simulink library "library"  (R2020a)
settings: Solver=VariableStepAuto  StartTime=0.0  StopTime=10.0  RelTol=1e-3
values from neighbouring files (symbols this model uses):
  height = 1080    [setup.m]    (also in setupSystem.m = heightName(nameIdx))
  nRho = maxRho*2    [setup.m]    (also in setupSystem.m)
  theta = (0:dTheta:180-dTheta)    [ARLHT.m]    (also in setup.m = (0:1:179); setupSystem.m = (0:1:179))
  width = 1920    [setup.m]    (also in setupSystem.m = widthName(nameIdx))
libraries: simulink x135, hdlsllib x83, $bdroot x15
(part 1 of 3)
settings Model: Creator=david  LastModifiedBy=david

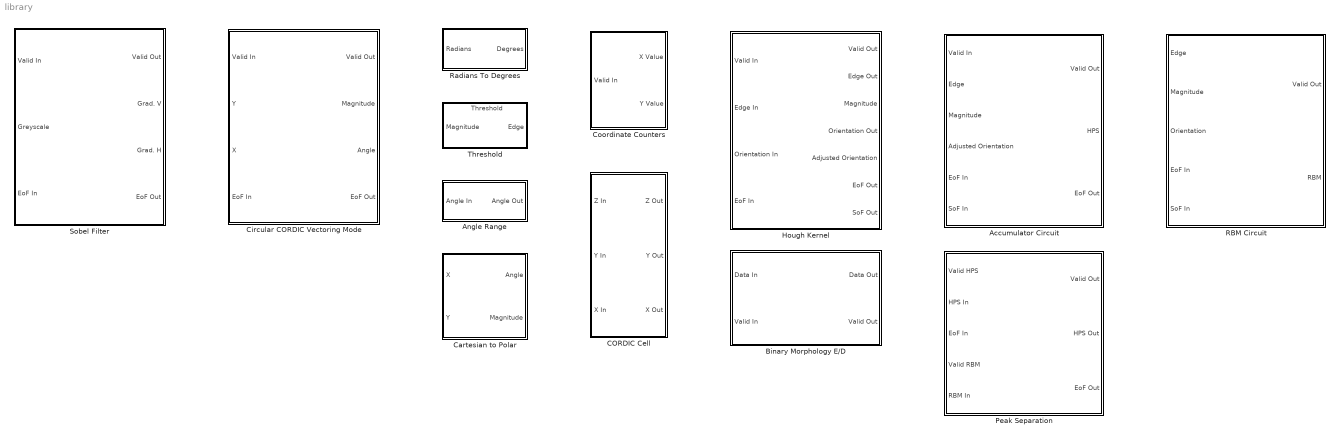
== system library ==
  Accumulator Circuit : Subsystem  mask{height=height, width=width, rhoBits=ceil(log2(ceil(sqrt(height^2+width^2)*4))), nTheta=length(theta), nRho=nRho}
      mask prompts: height "Image Height:"; width "Image Width:"; rhoBits "Address Bits:"; nTheta "Number Theta:"; nRho "Number Rho:"
      mask init:
      | kTheta = 4;
  Angle Range : Subsystem
  Binary Morphology E/D : Subsystem  mask{operation=Erosion, height=height, width=width}
      mask prompts: height "Image Height:"; width "Image Width:"
      mask init:
      | if get_param(gcb, 'operation') == "Erosion"
      |     op = 0;
      | else
      |     op = 1;
      | end
      mask TypeOptions operation: Erosion | Dilation
      mask DialogControl ParameterGroupVar Prompt: Main
  CORDIC Cell : Subsystem  mask{k=0}
      mask prompts: k "Iteration Number:"
  Cartesian to Polar : Subsystem  mask{b=16, f=8}
      mask prompts: b "Angle Wordlength:"; f "Angle Fractional Bits:"
      mask DialogControl DescGroupVar Prompt: Cartesian to Polar
      mask DialogControl DescTextVar Prompt: Convert cartesian coordinates to polar representation. This block uses Circular CORDIC operating in vectoring mode. The output angle is in the range [-90, 90] degrees.
      mask DialogControl ParameterGroupVar Prompt: Main
  Circular CORDIC Vectoring Mode : Subsystem  mask{i=12, b=24, f=13}
      mask prompts: i "Number of Iterations:"; b "Wordlength:"; f "Fractional Bits:"
      mask DialogControl DescGroupVar Prompt: Circular CORDIC Vectoring Mode
      mask DialogControl DescTextVar Prompt: Implements circular CORDIC operating in vectoring mode. Outputs magnitude of x and y inputs. Computes the angle in range [-pi, pi].
      mask DialogControl ParameterGroupVar Prompt: Main
  Coordinate Counters : Subsystem  mask{height=480, width=640}
      mask prompts: height "Image Height:"; width "Image Width:"
      mask DialogControl DescGroupVar Prompt: Coordinate Counters
      mask DialogControl DescTextVar Prompt: Coordinate HDL counters to keep track of coordinate values.
      mask DialogControl ParameterGroupVar Prompt: Main
  Hough Kernel : Subsystem  mask{rhoBits=ceil(log2(ceil(sqrt(height^2+width^2))*2)), height=height, width=width, dTheta=1}
      mask prompts: rhoBits "Address Bits:"; height "Image Height:"; width "Image Width:"; dTheta "Theta Resolution:"
      mask init:
      | kTheta = 4;
      | maxRho = ceil(sqrt((height/2)^2+(width/2)^2));
      | theta = (0:dTheta:180-dTheta);
      | gamma = (theta(end) + dTheta)/kTheta;
  Peak Separation : Subsystem  mask{nRho=ceil(sqrt(height^2+width^2))*2, nTheta=length(theta)}
      mask prompts: nRho "HPS Height:"; nTheta "HPS Width:"
      mask DialogControl DescGroupVar Prompt: Peak Separation
      mask DialogControl ParameterGroupVar Prompt: Main
  RBM Circuit : Subsystem  mask{height=height, width=width, nTheta=length(theta), rhoBits=ceil(log2(ceil(sqrt(height^2+width^2))*2)), nRho=nRho}
      mask prompts: height "Image Height:"; width "Image Width:"; nTheta "Number Theta:"; rhoBits "Address Bits:"; nRho "Number Rho:"
  Radians To Degrees : Subsystem  mask{f=0}
      mask prompts: f "Fractional Bits:"
      mask DialogControl DescGroupVar Prompt: Radian to Degrees
      mask DialogControl DescTextVar Prompt: Convert radians to degrees and output angle based on input resolution in degrees.
      mask DialogControl ParameterGroupVar Prompt: Main
  Sobel Filter : Subsystem  mask{height=height, width=width}
      mask prompts: height "Image Height:"; width "Image Width:"
      mask DialogControl DescGroupVar Prompt: Sobel Filter
      mask DialogControl DescTextVar Prompt: The Sobel Filter block applies the Sobel edge detection filters to a greyscale image to produce the horizontal and vertical gradients. The symmetric border management scheme is used in this block.
      mask DialogControl ParameterGroupVar Prompt: Main
  Threshold : Subsystem  mask{b=11, f=0, s=0}
      mask prompts: b "Wordlength:"; f "Fractional Bits:"; s "Signed:"
      settings: PortSchema="{\"entries\":[{\"content\":{\"sides\":[{\"content\":{\"connectorIds\":[\"In1\"]},\"type\":\"ConnectorPlacement.EquallySpacedRectSide\",\"uuid\":\"2eddfc8d-913f-4b03-9e43-0dfa341f5c16\"},{\"content\":{\"connectorIds\":[\"Out1\"],\"side\":\"RIGHT\"},\"type\":\"ConnectorPlacement.EquallySpacedRectSide\",\"uuid\":\"673922c3-77d1-427d-93a1-c0d3defe75f8\"},{\"content\":{\"connectorIds\":[\"In2\"],\"side\":\"TOP\"},\"type\":\"ConnectorPlacement.EquallySpacedRectSide\",\"uuid\":\"7679a1c8-69e5-4154-8188-f484296a7f7e\"}]},\"type\":\"ConnectorPlacement.EquallySpacedConnector\",\"uuid\":\"713163ba-a4f5-4467-a1a5-cd71dca6c6a2\"}],\"packageUris\":[\"http://schema.mathworks.com/mf0/Connector/19700101\"],\"version\":\"1.0\"}"
      mask DialogControl DescGroupVar Prompt: Threshold
      mask DialogControl DescTextVar Prompt: Segment an input signal using a threshold value.
      mask DialogControl ParameterGroupVar Prompt: Main

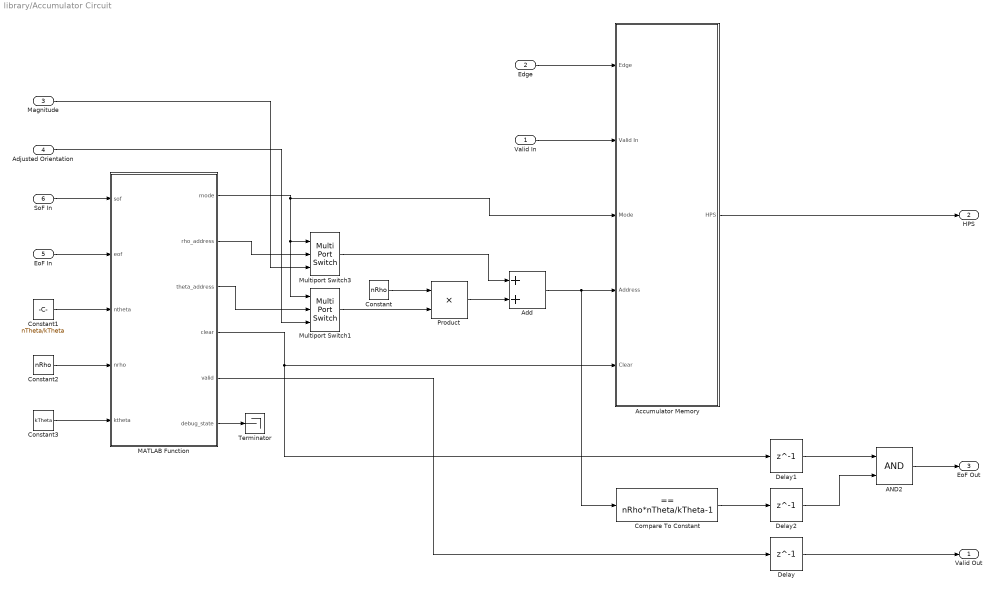
== system library/Accumulator Circuit ==
  Valid In : Inport
  Edge : Inport  Port=2
  Magnitude : Inport  Port=3
  Adjusted Orientation : Inport  Port=4
  EoF In : Inport  Port=5
  SoF In : Inport  Port=6
  AND2 : Logic  IconShape=distinctive  AllPortsSameDT=off  OutDataTypeStr=boolean
  Accumulator Memory : Subsystem
  Add : Sum  OutDataTypeStr=fixdt(0,ceil(log2(nRho*nTheta/kTheta)),0)
  Compare To Constant : simulink/Logic and Bit Operations/Compare To Constant  relop===  const=nRho*nTheta/kTheta-1  OutDataTypeStr=boolean
  Constant : Constant  Value=nRho  OutDataTypeStr=fixdt(0,ceil(log2(nRho+1)),0)  SampleTime=-1
  Constant1 : Constant  Value=nTheta/kTheta  OutDataTypeStr=uint8  SampleTime=-1
  Constant2 : Constant  Value=nRho  OutDataTypeStr=uint16  SampleTime=-1
  Constant3 : Constant  Value=kTheta  OutDataTypeStr=uint8  SampleTime=-1
  Delay : Delay  DelayLength=1  InitialCondition=0  UseCircularBuffer=on
  Delay1 : Delay  DelayLength=1  InitialCondition=0  UseCircularBuffer=on
  Delay2 : Delay  DelayLength=1  InitialCondition=0  UseCircularBuffer=on
  MATLAB Function : MATLAB Function  TreatAsAtomicUnit=on
  Multiport Switch1 : MultiPortSwitch  DataPortOrder=Zero-based contiguous  Inputs=2  zeroidx=on
  Multiport Switch3 : MultiPortSwitch  DataPortOrder=Zero-based contiguous  Inputs=2  zeroidx=on
  Product : Product  OutDataTypeStr=fixdt(0,ceil(log2(nRho*(nTheta/kTheta-1))),0)
  Terminator : Terminator
  Valid Out : Outport
  HPS : Outport  Port=2
  EoF Out : Outport  Port=3
  wires:
  EoF In/1 -> MATLAB Function/2(eof)
  MATLAB Function/3(theta_address) -> Multiport Switch1/2
  MATLAB Function/2(rho_address) -> Multiport Switch3/2
  MATLAB Function/1(mode) -> Accumulator Memory/3(Mode), Multiport Switch3/1, Multiport Switch1/1
  Constant/1 -> Product/1
  Product/1 -> Add/2
  Multiport Switch3/1 -> Add/1
  Multiport Switch1/1 -> Product/2
  Add/1 -> Accumulator Memory/4(Address), Compare To Constant/1
  Accumulator Memory/1(HPS) -> HPS/1
  Valid In/1 -> Accumulator Memory/2(Valid In)
  Edge/1 -> Accumulator Memory/1(Edge)
  Adjusted Orientation/1 -> Multiport Switch1/3
  Magnitude/1 -> Multiport Switch3/3
  Compare To Constant/1 -> Delay2/1
  Constant3/1 -> MATLAB Function/5(ktheta)
  Constant2/1 -> MATLAB Function/4(nrho)
  Constant1/1 -> MATLAB Function/3(ntheta)
  Delay2/1 -> AND2/2
  Delay1/1 -> AND2/1
  AND2/1 -> EoF Out/1
  Delay/1 -> Valid Out/1
  MATLAB Function/5(valid) -> Delay/1
  MATLAB Function/4(clear) -> Accumulator Memory/5(Clear), Delay1/1
  SoF In/1 -> MATLAB Function/1(sof)
  MATLAB Function/6(debug_state) -> Terminator/1

== system library/Angle Range ==
  Angle In : Inport
  Add : Sum  OutDataTypeStr=uint8
  Compare To Constant : simulink/Logic and Bit Operations/Compare To Constant  relop=<  const=0  OutDataTypeStr=boolean
  Constant : Constant  Value=180  OutDataTypeStr=uint8  SampleTime=-1
  Data Type Conversion : DataTypeConversion  OutDataTypeStr=uint8
  Multiport Switch : MultiPortSwitch  DataPortOrder=Zero-based contiguous  Inputs=2  zeroidx=on
  Angle Out : Outport
  wires:
  Constant/1 -> Add/2
  Add/1 -> Multiport Switch/3
  Data Type Conversion/1 -> Multiport Switch/2
  Compare To Constant/1 -> Multiport Switch/1
  Angle In/1 -> Compare To Constant/1, Data Type Conversion/1, Add/1
  Multiport Switch/1 -> Angle Out/1

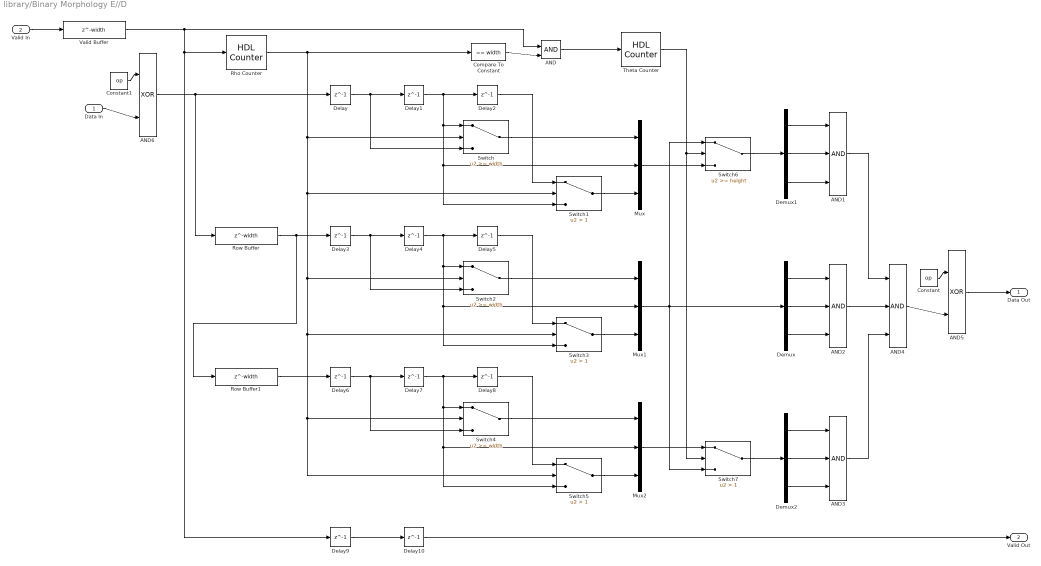
== system library/Binary Morphology E//D ==
  Data In : Inport
  Valid In : Inport  Port=2
  AND : Logic  IconShape=distinctive  AllPortsSameDT=off  OutDataTypeStr=boolean
  AND{1..4} (4 alike) : Logic  Inputs=3  IconShape=distinctive  AllPortsSameDT=off  OutDataTypeStr=boolean
  AND5 : Logic  Operator=XOR  IconShape=distinctive  AllPortsSameDT=off  OutDataTypeStr=boolean
  AND6 : Logic  Operator=XOR  IconShape=distinctive  AllPortsSameDT=off  OutDataTypeStr=boolean
  Compare To Constant : simulink/Logic and Bit Operations/Compare To Constant  relop===  const=width  OutDataTypeStr=boolean
  Constant : Constant  Value=op  OutDataTypeStr=Inherit: Inherit via back propagation  SampleTime=-1
  Constant1 : Constant  Value=op  OutDataTypeStr=Inherit: Inherit via back propagation  SampleTime=-1
  Delay{,1..10} (11 alike) : Delay  DelayLength=1
  Demux : Demux  Outputs=3
  Demux1 : Demux  Outputs=3
  Demux2 : Demux  Outputs=3
  Mux : Mux  Inputs=3
  Mux1 : Mux  Inputs=3
  Mux2 : Mux  Inputs=3
  Rho Counter : hdlsllib/Sources/HDL Counter  CountType=Count limited  CountInit=1  CountStep=1  CountMax=width  CountFromType=Initial value  CountFrom=1  CountResetPort=off  CountLoadPort=off  CountEnbPort=on  CountDirPort=off  CountDataType=Unsigned  CountWordLen=ceil(log2(width+1))  CountFracLen=0  CountSampTime=1
  Row Buffer : Delay  DelayLength=width
  Row Buffer1 : Delay  DelayLength=width
  Switch : Switch  Threshold=width
  Switch{1,3,5,7} (4 alike) : Switch  Criteria=u2 > Threshold  Threshold=1
  Switch2 : Switch  Threshold=width
  Switch4 : Switch  Threshold=width
  Switch6 : Switch  Threshold=height
  Theta Counter : hdlsllib/Sources/HDL Counter  CountType=Count limited  CountInit=1  CountStep=1  CountMax=height  CountFromType=Initial value  CountFrom=1  CountResetPort=off  CountLoadPort=off  CountEnbPort=on  CountDirPort=off  CountDataType=Unsigned  CountWordLen=ceil(log2(height+1))  CountFracLen=0  CountSampTime=1
  Valid Buffer : Delay  DelayLength=width
  Data Out : Outport
  Valid Out : Outport  Port=2
  wires:
  Data In/1 -> AND6/2
  AND6/1 -> Delay/1, Row Buffer/1
  Constant1/1 -> AND6/1
  Constant/1 -> AND5/1
  AND4/1 -> AND5/2
  AND3/1 -> AND4/3
  AND1/1 -> AND4/1
  AND2/1 -> AND4/2
  Demux2/3 -> AND3/3
  Demux2/1 -> AND3/1
  Demux2/2 -> AND3/2
  Demux/3 -> AND2/3
  Demux/2 -> AND2/2
  Demux/1 -> AND2/1
  Demux1/3 -> AND1/3
  Demux1/1 -> AND1/1
  Demux1/2 -> AND1/2
  Switch7/1 -> Demux2/1
  Mux2/1 -> Switch7/1
  Mux/1 -> Switch6/3
  Theta Counter/1 -> Switch6/2, Switch7/2
  Switch6/1 -> Demux1/1
  Mux1/1 -> Demux/1, Switch6/1, Switch7/3
  Row Buffer1/1 -> Delay6/1
  Rho Counter/1 -> Compare To Constant/1, Switch/2, Switch1/2, Switch2/2, Switch5/2, Switch4/2, Switch3/2
  Switch5/1 -> Mux2/3
  Switch4/1 -> Mux2/1
  Delay8/1 -> Switch5/1
  Delay7/1 -> Switch4/1, Switch5/3, Mux2/2, Delay8/1
  Delay6/1 -> Delay7/1, Switch4/3
  Delay3/1 -> Switch2/3, Delay4/1
  Delay4/1 -> Delay5/1, Mux1/2, Switch3/3, Switch2/1
  Delay5/1 -> Switch3/1
  Switch2/1 -> Mux1/1
  Switch3/1 -> Mux1/3
  Row Buffer/1 -> Row Buffer1/1, Delay3/1
  Switch1/1 -> Mux/3
  Switch/1 -> Mux/1
  Delay2/1 -> Switch1/1
  Delay1/1 -> Switch/1, Switch1/3, Mux/2, Delay2/1
  Delay/1 -> Delay1/1, Switch/3
  Compare To Constant/1 -> AND/2
  AND/1 -> Theta Counter/1
  Valid In/1 -> Valid Buffer/1
  Valid Buffer/1 -> Rho Counter/1, Delay9/1, AND/1
  Delay9/1 -> Delay10/1
  Delay10/1 -> Valid Out/1
  AND5/1 -> Data Out/1

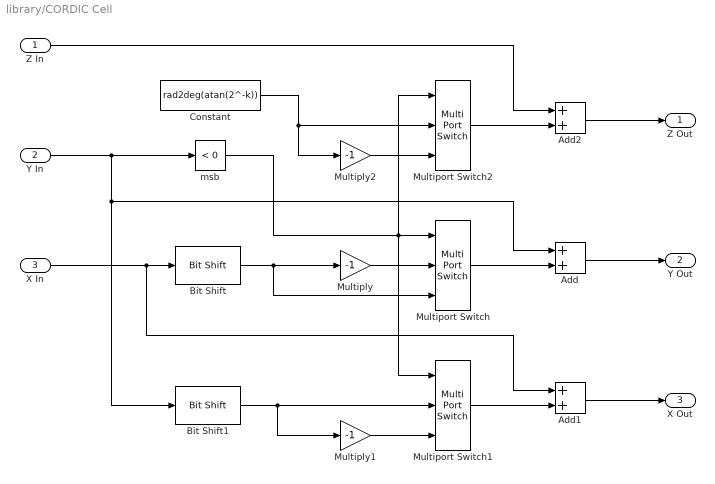
== system library/CORDIC Cell ==
  Z In : Inport
  Y In : Inport  Port=2
  X In : Inport  Port=3
  Add : Sum  RndMeth=Round  SaturateOnIntegerOverflow=on  OutDataTypeStr=Inherit: Same as first input
  Add1 : Sum  RndMeth=Round  SaturateOnIntegerOverflow=on  OutDataTypeStr=Inherit: Same as first input
  Add2 : Sum  RndMeth=Round  SaturateOnIntegerOverflow=on  OutDataTypeStr=Inherit: Same as first input
  Bit Shift : hdlsllib/Logic and Bit Operations/Bit Shift  mode=Shift Right Arithmetic  N=k
  Bit Shift1 : hdlsllib/Logic and Bit Operations/Bit Shift  mode=Shift Right Arithmetic  N=k
  Constant : Constant  Value=rad2deg(atan(2^-k))  OutDataTypeStr=Inherit: Inherit via back propagation  SampleTime=-1
  Multiply : Gain  Gain=-1  OutDataTypeStr=Inherit: Same as input
  Multiply1 : Gain  Gain=-1  OutDataTypeStr=Inherit: Same as input
  Multiply2 : Gain  Gain=-1  OutDataTypeStr=Inherit: Same as input
  Multiport Switch : MultiPortSwitch  DataPortOrder=Zero-based contiguous  Inputs=2  zeroidx=on
  Multiport Switch1 : MultiPortSwitch  DataPortOrder=Zero-based contiguous  Inputs=2  zeroidx=on
  Multiport Switch2 : MultiPortSwitch  DataPortOrder=Zero-based contiguous  Inputs=2  zeroidx=on
  msb : simulink/Logic and Bit Operations/Compare To Constant  relop=<  const=0  OutDataTypeStr=boolean
  Z Out : Outport
  Y Out : Outport  Port=2
  X Out : Outport  Port=3
  wires:
  Multiply1/1 -> Multiport Switch1/3
  Multiply/1 -> Multiport Switch/2
  Add/1 -> Y Out/1
  Add1/1 -> X Out/1
  Add2/1 -> Z Out/1
  Multiport Switch/1 -> Add/2
  Multiport Switch1/1 -> Add1/2
  X In/1 -> Bit Shift/1, Add1/1
  Bit Shift1/1 -> Multiply1/1, Multiport Switch1/2
  Bit Shift/1 -> Multiply/1, Multiport Switch/3
  msb/1 -> Multiport Switch/1, Multiport Switch1/1, Multiport Switch2/1
  Y In/1 -> msb/1, Bit Shift1/1, Add/1
  Z In/1 -> Add2/1
  Multiply2/1 -> Multiport Switch2/3
  Constant/1 -> Multiply2/1, Multiport Switch2/2
  Multiport Switch2/1 -> Add2/2

== system library/Cartesian to Polar ==
  X : Inport
  Y : Inport  Port=2
  CORDIC Cells : Subsystem
  Compare To Zero : simulink/Logic and Bit Operations/Compare To Zero  relop=~=  OutDataTypeStr=boolean
  Gain : Gain  Gain=1/1.6467  ParamDataTypeStr=fixdt(0,16,16)  RndMeth=Round  SaturateOnIntegerOverflow=on  OutDataTypeStr=Inherit: Same as input
  Multiport Switch : MultiPortSwitch  DataPortOrder=Zero-based contiguous  Inputs=2  zeroidx=on
  Quadrant Demapper : Subsystem
  Quadrant Mapper : Subsystem
  Terminator : Terminator
  Z : Constant  Value=0  OutDataTypeStr=fixdt(1,b,f)  SampleTime=-1
  Angle : Outport
  Magnitude : Outport  Port=2
  wires:
  Quadrant Demapper/1(Z Out) -> Multiport Switch/3
  Multiport Switch/1 -> Angle/1
  Y/1 -> Quadrant Mapper/1(Y In)
  X/1 -> Quadrant Mapper/2(X In)
  Gain/1 -> Magnitude/1
  Compare To Zero/1 -> Multiport Switch/1
  CORDIC Cells/1(Z Out) -> Quadrant Demapper/1(Z In)
  Quadrant Mapper/3(Decision) -> Quadrant Demapper/2(Decision)
  CORDIC Cells/2(Y Out) -> Terminator/1
  CORDIC Cells/3(X Out) -> Gain/1
  Z/1 -> CORDIC Cells/1(Z In), Multiport Switch/2
  Quadrant Mapper/2(X Out) -> CORDIC Cells/3(X In)
  Quadrant Mapper/1(Y Out) -> CORDIC Cells/2(Y In), Compare To Zero/1

== system library/Circular CORDIC Vectoring Mode ==
  Valid In : Inport
  Y : Inport  Port=2
  X : Inport  Port=3
  EoF In : Inport  Port=4
  Cartesian to Polar : $bdroot/Cartesian to Polar  b=16  f=8
  Data Type Conversion : DataTypeConversion  OutDataTypeStr=fixdt(1,24,11)
  Data Type Conversion1 : DataTypeConversion  OutDataTypeStr=fixdt(1,24,11)
  Valid Out : Outport  VectorParamsAs1DForOutWhenUnconnected=off
  Magnitude : Outport  Port=2  VectorParamsAs1DForOutWhenUnconnected=off
  Angle : Outport  Port=3  VectorParamsAs1DForOutWhenUnconnected=off
  EoF Out : Outport  Port=4  VectorParamsAs1DForOutWhenUnconnected=off
  wires:
  Valid In/1 -> Valid Out/1
  Cartesian to Polar/1 -> Angle/1
  Cartesian to Polar/2 -> Magnitude/1
  EoF In/1 -> EoF Out/1
  X/1 -> Data Type Conversion/1
  Y/1 -> Data Type Conversion1/1
  Data Type Conversion/1 -> Cartesian to Polar/1
  Data Type Conversion1/1 -> Cartesian to Polar/2

== system library/Coordinate Counters ==
  Valid In : Inport
  AND : Logic  IconShape=distinctive  AllPortsSameDT=off  OutDataTypeStr=boolean
  Compare To Constant : simulink/Logic and Bit Operations/Compare To Constant  relop===  const=width/2-1  OutDataTypeStr=boolean
  X Counter : hdlsllib/Sources/HDL Counter  CountType=Count limited  CountInit=-width/2  CountStep=1  CountMax=width/2-1  CountFromType=Initial value  CountFrom=-width/2  CountResetPort=off  CountLoadPort=off  CountEnbPort=on  CountDirPort=off  CountDataType=Signed  CountWordLen=ceil(log2(width/2)) + 1  CountFracLen=0  CountSampTime=1
  Y Counter : hdlsllib/Sources/HDL Counter  CountType=Count limited  CountInit=-height/2  CountStep=1  CountMax=height/2-1  CountFromType=Initial value  CountFrom=-height/2  CountResetPort=off  CountLoadPort=off  CountEnbPort=on  CountDirPort=off  CountDataType=Signed  CountWordLen=ceil(log2(height/2)) + 1  CountFracLen=0  CountSampTime=1
  X Value : Outport  VectorParamsAs1DForOutWhenUnconnected=off
  Y Value : Outport  Port=2  VectorParamsAs1DForOutWhenUnconnected=off
  wires:
  Valid In/1 -> AND/2, X Counter/1
  X Counter/1 -> X Value/1, Compare To Constant/1
  Y Counter/1 -> Y Value/1
  AND/1 -> Y Counter/1
  Compare To Constant/1 -> AND/1

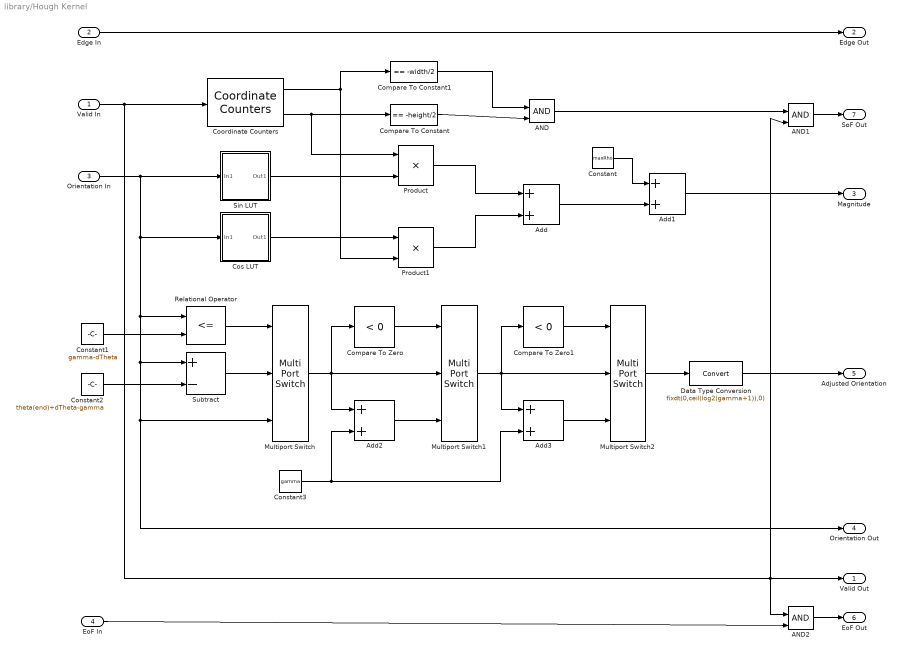
== system library/Hough Kernel ==
  Valid In : Inport
  Edge In : Inport  Port=2
  Orientation In : Inport  Port=3
  EoF In : Inport  Port=4
  AND : Logic  IconShape=distinctive  AllPortsSameDT=off  OutDataTypeStr=boolean
  AND1 : Logic  IconShape=distinctive  AllPortsSameDT=off  OutDataTypeStr=boolean
  AND2 : Logic  IconShape=distinctive  AllPortsSameDT=off  OutDataTypeStr=boolean
  Add : Sum
  Add1 : Sum  OutDataTypeStr=fixdt(0,rhoBits,0)
  Add2 : Sum  OutDataTypeStr=Inherit: Same as first input
  Add3 : Sum  OutDataTypeStr=Inherit: Same as first input
  Compare To Constant : simulink/Logic and Bit Operations/Compare To Constant  relop===  const=-height/2  OutDataTypeStr=boolean
  Compare To Constant1 : simulink/Logic and Bit Operations/Compare To Constant  relop===  const=-width/2  OutDataTypeStr=boolean
  Compare To Zero : simulink/Logic and Bit Operations/Compare To Zero  relop=<  OutDataTypeStr=boolean
  Compare To Zero1 : simulink/Logic and Bit Operations/Compare To Zero  relop=<  OutDataTypeStr=boolean
  Constant : Constant  Value=maxRho  OutDataTypeStr=fixdt(0,ceil(log2(maxRho+1)),0)  SampleTime=-1
  Constant1 : Constant  Value=gamma-dTheta  OutDataTypeStr=fixdt(0,ceil(log2(gamma)),0)  SampleTime=-1
  Constant2 : Constant  Value=theta(end)+dTheta-gamma  OutDataTypeStr=fixdt(0,ceil(log2(179+1-gamma)),0)  SampleTime=-1
  Constant3 : Constant  Value=gamma  OutDataTypeStr=fixdt(0,ceil(log2(gamma+1)),0)  SampleTime=-1
  Coordinate Counters : $bdroot/Coordinate Counters  height=height  width=width
  Cos LUT : Subsystem
  Data Type Conversion : DataTypeConversion  OutDataTypeStr=fixdt(0,ceil(log2(gamma+1)),0)
  Multiport Switch : MultiPortSwitch  DataPortOrder=Zero-based contiguous  Inputs=2  zeroidx=on
  Multiport Switch1 : MultiPortSwitch  DataPortOrder=Zero-based contiguous  Inputs=2  zeroidx=on
  Multiport Switch2 : MultiPortSwitch  DataPortOrder=Zero-based contiguous  Inputs=2  zeroidx=on
  Product : Product  OutDataTypeStr=fixdt(1,ceil(log2(height)),0)  RndMeth=Round
  Product1 : Product  OutDataTypeStr=fixdt(1,ceil(log2(width)),0)  RndMeth=Round
  Relational Operator : RelationalOperator  Operator=<=  OutDataTypeStr=boolean  RndMeth=Simplest
  Sin LUT : Subsystem
  Subtract : Sum  Inputs=+-  OutDataTypeStr=fixdt(1,9,0)
  Valid Out : Outport
  Edge Out : Outport  Port=2
  Magnitude : Outport  Port=3
  Orientation Out : Outport  Port=4
  Adjusted Orientation : Outport  Port=5
  EoF Out : Outport  Port=6
  SoF Out : Outport  Port=7
  wires:
  Edge In/1 -> Edge Out/1
  Coordinate Counters/2 -> Product/1, Compare To Constant/1
  Coordinate Counters/1 -> Product1/2, Compare To Constant1/1
  Product1/1 -> Add/2
  Constant/1 -> Add1/1
  Relational Operator/1 -> Multiport Switch/1
  Add/1 -> Add1/2
  Constant3/1 -> Add3/2, Add2/2
  Constant2/1 -> Subtract/2
  Add3/1 -> Multiport Switch2/3
  Add2/1 -> Multiport Switch1/3
  Add1/1 -> Magnitude/1
  Subtract/1 -> Multiport Switch/2
  Product/1 -> Add/1
  Compare To Zero1/1 -> Multiport Switch2/1
  Multiport Switch/1 -> Add2/1, Compare To Zero/1, Multiport Switch1/2
  Multiport Switch1/1 -> Add3/1, Compare To Zero1/1, Multiport Switch2/2
  Compare To Zero/1 -> Multiport Switch1/1
  Orientation In/1 -> Sin LUT/1(In1), Cos LUT/1(In1), Multiport Switch/3, Orientation Out/1, Subtract/1, Relational Operator/1
  Multiport Switch2/1 -> Data Type Conversion/1
  Constant1/1 -> Relational Operator/2
  Data Type Conversion/1 -> Adjusted Orientation/1
  Compare To Constant1/1 -> AND/1
  Compare To Constant/1 -> AND/2
  AND1/1 -> SoF Out/1
  AND/1 -> AND1/1
  Valid In/1 -> AND2/1, AND1/2, Valid Out/1, Coordinate Counters/1
  AND2/1 -> EoF Out/1
  EoF In/1 -> AND2/2
  Cos LUT/1(Out1) -> Product1/1
  Sin LUT/1(Out1) -> Product/2

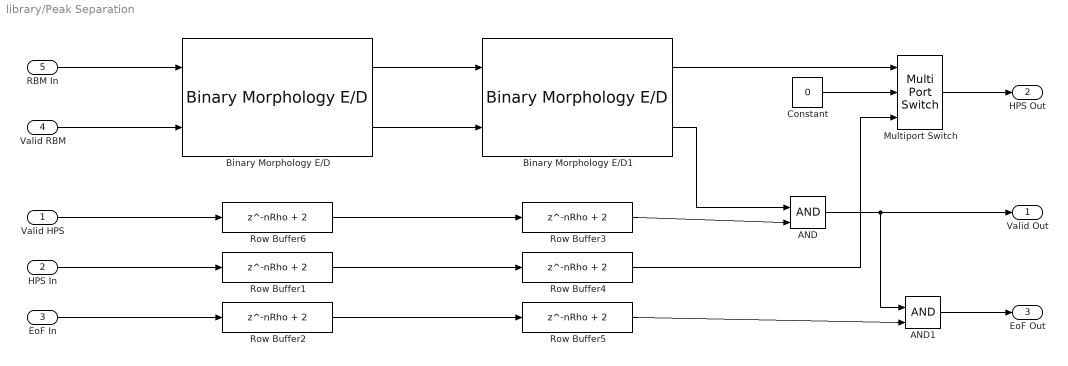
== system library/Peak Separation ==
  Valid HPS : Inport
  HPS In : Inport  Port=2
  EoF In : Inport  Port=3
  Valid RBM : Inport  Port=4
  RBM In : Inport  Port=5
  AND : Logic  IconShape=distinctive  AllPortsSameDT=off  OutDataTypeStr=boolean
  AND1 : Logic  IconShape=distinctive  AllPortsSameDT=off  OutDataTypeStr=boolean
  Binary Morphology E/D : $bdroot/Binary Morphology E//D  operation=Erosion  height=nTheta  width=nRho
  Binary Morphology E/D1 : $bdroot/Binary Morphology E//D  operation=Dilation  height=nTheta  width=nRho
  Constant : Constant  Value=0  OutDataTypeStr=Inherit: Inherit via back propagation  SampleTime=-1
  Multiport Switch : MultiPortSwitch  DataPortOrder=Zero-based contiguous  Inputs=2  zeroidx=on
  Row Buffer{1..6} (6 alike) : Delay  DelayLength=nRho + 2
  Valid Out : Outport
  HPS Out : Outport  Port=2
  EoF Out : Outport  Port=3
  wires:
  Row Buffer6/1 -> Row Buffer3/1
  Row Buffer2/1 -> Row Buffer5/1
  Row Buffer1/1 -> Row Buffer4/1
  Constant/1 -> Multiport Switch/2
  Row Buffer3/1 -> AND/2
  Binary Morphology E/D1/2 -> AND/1
  Valid HPS/1 -> Row Buffer6/1
  HPS In/1 -> Row Buffer1/1
  EoF In/1 -> Row Buffer2/1
  RBM In/1 -> Binary Morphology E/D/1
  Valid RBM/1 -> Binary Morphology E/D/2
  Binary Morphology E/D/1 -> Binary Morphology E/D1/1
  Binary Morphology E/D/2 -> Binary Morphology E/D1/2
  Binary Morphology E/D1/1 -> Multiport Switch/1
  Row Buffer4/1 -> Multiport Switch/3
  Multiport Switch/1 -> HPS Out/1
  AND1/1 -> EoF Out/1
  AND/1 -> AND1/1, Valid Out/1
  Row Buffer5/1 -> AND1/2

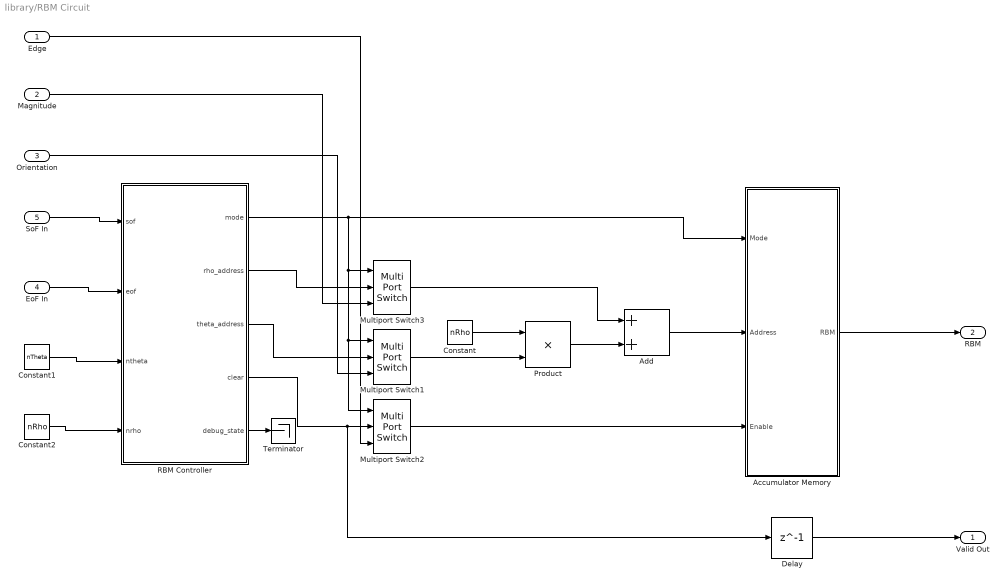
== system library/RBM Circuit ==
  Edge : Inport
  Magnitude : Inport  Port=2
  Orientation : Inport  Port=3
  EoF In : Inport  Port=4
  SoF In : Inport  Port=5
  Accumulator Memory : Subsystem
  Add : Sum  OutDataTypeStr=fixdt(0,ceil(log2(nRho*nTheta)),0)
  Constant : Constant  Value=nRho  OutDataTypeStr=fixdt(0,ceil(log2(nRho+1)),0)  SampleTime=-1
  Constant1 : Constant  Value=nTheta  OutDataTypeStr=uint8  SampleTime=-1
  Constant2 : Constant  Value=nRho  OutDataTypeStr=uint16  SampleTime=-1
  Delay : Delay  DelayLength=1  InitialCondition=0  UseCircularBuffer=on
  Multiport Switch1 : MultiPortSwitch  DataPortOrder=Zero-based contiguous  Inputs=2  zeroidx=on
  Multiport Switch2 : MultiPortSwitch  DataPortOrder=Zero-based contiguous  Inputs=2  zeroidx=on
  Multiport Switch3 : MultiPortSwitch  DataPortOrder=Zero-based contiguous  Inputs=2  zeroidx=on
  Product : Product  OutDataTypeStr=fixdt(0,ceil(log2(nRho*(nTheta))),0)
  RBM Controller : MATLAB Function  TreatAsAtomicUnit=on
  Terminator : Terminator
  Valid Out : Outport
  RBM : Outport  Port=2
  wires:
  EoF In/1 -> RBM Controller/2(eof)
  Multiport Switch2/1 -> Accumulator Memory/3(Enable)
  Edge/1 -> Multiport Switch2/3
  SoF In/1 -> RBM Controller/1(sof)
  RBM Controller/4(clear) -> Delay/1, Multiport Switch2/2
  Delay/1 -> Valid Out/1
  Constant1/1 -> RBM Controller/3(ntheta)
  Constant2/1 -> RBM Controller/4(nrho)
  Magnitude/1 -> Multiport Switch3/3
  Orientation/1 -> Multiport Switch1/3
  Accumulator Memory/1(RBM) -> RBM/1
  Add/1 -> Accumulator Memory/2(Address)
  Multiport Switch1/1 -> Product/2
  Multiport Switch3/1 -> Add/1
  Product/1 -> Add/2
  Constant/1 -> Product/1
  RBM Controller/1(mode) -> Accumulator Memory/1(Mode), Multiport Switch1/1, Multiport Switch2/1, Multiport Switch3/1
  RBM Controller/2(rho_address) -> Multiport Switch3/2
  RBM Controller/3(theta_address) -> Multiport Switch1/2
  RBM Controller/5(debug_state) -> Terminator/1

== system library/Radians To Degrees ==
  Radians : Inport
  Data Type Conversion : DataTypeConversion  OutDataTypeStr=fixdt(1,9+f,f)  RndMeth=Round  SaturateOnIntegerOverflow=on
  Gain : Gain  Gain=1/pi  RndMeth=Round  SaturateOnIntegerOverflow=on  OutDataTypeStr=Inherit: Same as input  ParamDataTypeStr=Inherit: Same as input
  Gain1 : Gain  Gain=180  ParamDataTypeStr=uint8  RndMeth=Round  SaturateOnIntegerOverflow=on
  Degrees : Outport
  wires:
  Gain1/1 -> Data Type Conversion/1
  Gain/1 -> Gain1/1
  Data Type Conversion/1 -> Degrees/1
  Radians/1 -> Gain/1

== system library/Sobel Filter ==
  Valid In : Inport
  Greyscale : Inport  Port=2
  EoF In : Inport  Port=3
  Coordinate Counters : Subsystem
  Row Buffer : Delay  DelayLength=width
  Sobel Filter : Subsystem
  Valid Out : Outport  VectorParamsAs1DForOutWhenUnconnected=off
  Grad. V : Outport  Port=2  VectorParamsAs1DForOutWhenUnconnected=off
  Grad. H : Outport  Port=3  VectorParamsAs1DForOutWhenUnconnected=off
  EoF Out : Outport  Port=4  VectorParamsAs1DForOutWhenUnconnected=off
  wires:
  Sobel Filter/2(Gradient X) -> Grad. H/1
  Sobel Filter/1(Gradient Y) -> Grad. V/1
  Coordinate Counters/1(X Value) -> Sobel Filter/1(X Value)
  Valid In/1 -> Row Buffer/1
  Greyscale/1 -> Sobel Filter/3(Grayscale)
  Row Buffer/1 -> Sobel Filter/4(Valid In), Coordinate Counters/1(Valid In)
  EoF In/1 -> Sobel Filter/5(EoF In)
  Sobel Filter/3(Valid Out) -> Valid Out/1
  Sobel Filter/4(EoF Out) -> EoF Out/1
  Coordinate Counters/2(Y Value) -> Sobel Filter/2(Y Value)

== system library/Threshold ==
  Magnitude : Inport
  Threshold : Inport  Port=2
  Bit Shift : hdlsllib/Logic and Bit Operations/Bit Shift  mode=Shift Right Logical  N=2
  Data Type Conversion : DataTypeConversion  OutDataTypeStr=fixdt(s,b+f,f)  RndMeth=Round  SaturateOnIntegerOverflow=on
  Data Type Conversion1 : DataTypeConversion  OutDataTypeStr=fixdt(0,8,0)  SaturateOnIntegerOverflow=on
  Relational Operator : RelationalOperator  OutDataTypeStr=boolean  RndMeth=Simplest
  Edge : Outport
  wires:
  Magnitude/1 -> Data Type Conversion/1
  Data Type Conversion1/1 -> Relational Operator/1
  Threshold/1 -> Relational Operator/2
  Relational Operator/1 -> Edge/1
  Data Type Conversion/1 -> Bit Shift/1
  Bit Shift/1 -> Data Type Conversion1/1

== system library/Accumulator Circuit/Accumulator Memory ==
  Edge : Inport
  Valid In : Inport  Port=2
  Mode : Inport  Port=3
  Address : Inport  Port=4
  Clear : Inport  Port=5
  AND1 : Logic  IconShape=distinctive  AllPortsSameDT=off  OutDataTypeStr=boolean
  Accumulator Memory : Subsystem
  Multiport Switch2 : MultiPortSwitch  DataPortOrder=Zero-based contiguous  Inputs=2  zeroidx=on
  HPS : Outport
  wires:
  Clear/1 -> Multiport Switch2/2
  Edge/1 -> AND1/1
  AND1/1 -> Multiport Switch2/3
  Accumulator Memory/1(HPS) -> HPS/1
  Valid In/1 -> AND1/2
  Address/1 -> Accumulator Memory/2(Address)
  Multiport Switch2/1 -> Accumulator Memory/3(Enable)
  Mode/1 -> Accumulator Memory/1(Mode), Multiport Switch2/1

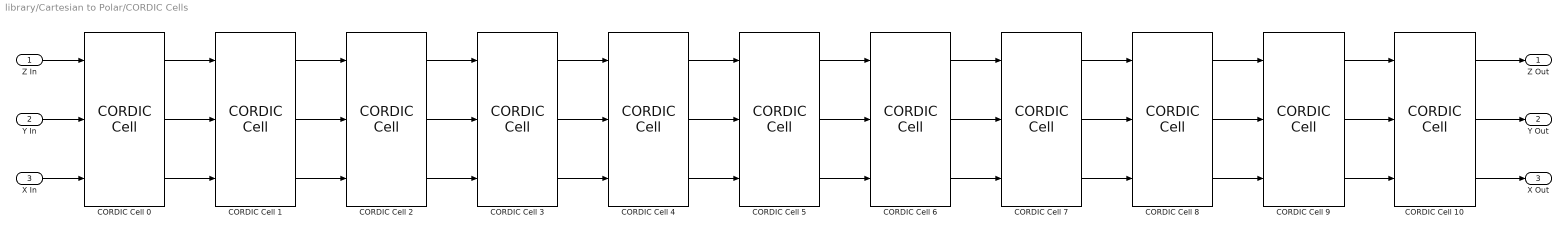
== system library/Cartesian to Polar/CORDIC Cells ==
  Z In : Inport
  Y In : Inport  Port=2
  X In : Inport  Port=3
  CORDIC Cell 0 : $bdroot/CORDIC Cell  k=0
  CORDIC Cell 1 : $bdroot/CORDIC Cell  k=1
  CORDIC Cell 10 : $bdroot/CORDIC Cell  k=10
  CORDIC Cell 2 : $bdroot/CORDIC Cell  k=2
  CORDIC Cell 3 : $bdroot/CORDIC Cell  k=3
  CORDIC Cell 4 : $bdroot/CORDIC Cell  k=4
  CORDIC Cell 5 : $bdroot/CORDIC Cell  k=5
  CORDIC Cell 6 : $bdroot/CORDIC Cell  k=6
  CORDIC Cell 7 : $bdroot/CORDIC Cell  k=7
  CORDIC Cell 8 : $bdroot/CORDIC Cell  k=8
  CORDIC Cell 9 : $bdroot/CORDIC Cell  k=9
  Z Out : Outport
  Y Out : Outport  Port=2
  X Out : Outport  Port=3
  wires:
  CORDIC Cell 10/3 -> X Out/1
  CORDIC Cell 10/2 -> Y Out/1
  CORDIC Cell 10/1 -> Z Out/1
  CORDIC Cell 9/1 -> CORDIC Cell 10/1
  CORDIC Cell 9/3 -> CORDIC Cell 10/3
  CORDIC Cell 9/2 -> CORDIC Cell 10/2
  CORDIC Cell 8/1 -> CORDIC Cell 9/1
  CORDIC Cell 8/3 -> CORDIC Cell 9/3
  CORDIC Cell 8/2 -> CORDIC Cell 9/2
  CORDIC Cell 7/1 -> CORDIC Cell 8/1
  CORDIC Cell 7/2 -> CORDIC Cell 8/2
  CORDIC Cell 7/3 -> CORDIC Cell 8/3
  CORDIC Cell 6/1 -> CORDIC Cell 7/1
  CORDIC Cell 6/2 -> CORDIC Cell 7/2
  CORDIC Cell 6/3 -> CORDIC Cell 7/3
  CORDIC Cell 5/3 -> CORDIC Cell 6/3
  CORDIC Cell 5/1 -> CORDIC Cell 6/1
  CORDIC Cell 5/2 -> CORDIC Cell 6/2
  CORDIC Cell 4/3 -> CORDIC Cell 5/3
  CORDIC Cell 4/1 -> CORDIC Cell 5/1
  CORDIC Cell 4/2 -> CORDIC Cell 5/2
  CORDIC Cell 3/1 -> CORDIC Cell 4/1
  CORDIC Cell 3/3 -> CORDIC Cell 4/3
  CORDIC Cell 3/2 -> CORDIC Cell 4/2
  CORDIC Cell 2/3 -> CORDIC Cell 3/3
  CORDIC Cell 2/1 -> CORDIC Cell 3/1
  CORDIC Cell 2/2 -> CORDIC Cell 3/2
  CORDIC Cell 1/1 -> CORDIC Cell 2/1
  CORDIC Cell 1/2 -> CORDIC Cell 2/2
  CORDIC Cell 1/3 -> CORDIC Cell 2/3
  CORDIC Cell 0/3 -> CORDIC Cell 1/3
  CORDIC Cell 0/1 -> CORDIC Cell 1/1
  CORDIC Cell 0/2 -> CORDIC Cell 1/2
  Z In/1 -> CORDIC Cell 0/1
  X In/1 -> CORDIC Cell 0/3
  Y In/1 -> CORDIC Cell 0/2

== system library/Cartesian to Polar/Quadrant Demapper ==
  Z In : Inport
  Decision : Inport  Port=2
  Add : Sum  Inputs=+-  OutDataTypeStr=Inherit: Same as first input
  Add1 : Sum  OutDataTypeStr=Inherit: Same as first input
  Constant : Constant  Value=90  OutDataTypeStr=uint8  SampleTime=-1
  Multiport Switch : MultiPortSwitch  DataPortOrder=Zero-based contiguous  Inputs=4  zeroidx=on
  Z Out : Outport
  wires:
  Add1/1 -> Multiport Switch/5
  Constant/1 -> Add/2, Add1/2
  Add/1 -> Multiport Switch/3
  Z In/1 -> Multiport Switch/2, Multiport Switch/4, Add/1, Add1/1
  Multiport Switch/1 -> Z Out/1
  Decision/1 -> Multiport Switch/1

== system library/Cartesian to Polar/Quadrant Mapper ==
  Y In : Inport
  X In : Inport  Port=2
  Bit Concat : hdlsllib/Logic and Bit Operations/Bit Concat  numInputs=2
  Compare To Zero : simulink/Logic and Bit Operations/Compare To Zero  relop=<  OutDataTypeStr=boolean
  Compare To Zero1 : simulink/Logic and Bit Operations/Compare To Zero  relop=<  OutDataTypeStr=boolean
  Gain : Gain  Gain=-1  OutDataTypeStr=Inherit: Same as input
  Gain1 : Gain  Gain=-1  OutDataTypeStr=Inherit: Same as input
  Multiport Switch : MultiPortSwitch  DataPortOrder=Zero-based contiguous  Inputs=4  zeroidx=on
  Multiport Switch1 : MultiPortSwitch  DataPortOrder=Zero-based contiguous  Inputs=4  zeroidx=on
  Y Out : Outport
  X Out : Outport  Port=2
  Decision : Outport  Port=3
  wires:
  Y In/1 -> Gain1/1, Multiport Switch1/4, Multiport Switch1/2, Multiport Switch/3, Compare To Zero1/1
  Gain1/1 -> Multiport Switch/5
  Gain/1 -> Multiport Switch1/3
  Multiport Switch1/1 -> Y Out/1
  Multiport Switch/1 -> X Out/1
  Bit Concat/1 -> Multiport Switch/1, Multiport Switch1/1, Decision/1
  Compare To Zero/1 -> Bit Concat/2
  Compare To Zero1/1 -> Bit Concat/1
  X In/1 -> Multiport Switch/4, Gain/1, Multiport Switch1/5, Multiport Switch/2, Compare To Zero/1

== system library/Hough Kernel/Cos LUT ==
  In1 : Inport
  Cos LUT : Lookup_n-D  NumberOfTableDimensions=1  BreakpointsForDimension1=theta  IndexSearchMethod=Evenly spaced points  Table=cos(deg2rad(theta))  InterpMethod=Flat  DiagnosticForOutOfRangeInput=Error  InternalRulePriority=Speed  OutDataTypeStr=fixdt(1,16,14)  RndMeth=Simplest  InputSameDT=on
  Out1 : Outport
  wires:
  In1/1 -> Cos LUT/1
  Cos LUT/1 -> Out1/1

== system library/Hough Kernel/Sin LUT ==
  In1 : Inport
  Sin LUT : Lookup_n-D  NumberOfTableDimensions=1  BreakpointsForDimension1=theta  IndexSearchMethod=Evenly spaced points  Table=sin(deg2rad(theta))  InterpMethod=Flat  DiagnosticForOutOfRangeInput=Error  InternalRulePriority=Speed  OutDataTypeStr=fixdt(1,16,14)  RndMeth=Simplest  InputSameDT=on
  Out1 : Outport
  wires:
  Sin LUT/1 -> Out1/1
  In1/1 -> Sin LUT/1
